simulink model "Powertrain_Performance_Design"  (R2024a)
settings: Solver=ode4  StartTime=0.0  StopTime=simtime  FixedStep=1  MaxStep=0.1  RelTol=1e-3
model workspace (MAT data in the model file):
  A_max = 2.22
  C_d = 0.23
  C_r = 0.011
  Cpack = 216
  DOD = [0 0.1 0.2 0.3 0.4 0.5 0.6 0.7 0.8 0.9 1 1.1 ... (1001 elements, 1001x1)]
  EM_N = [0 100 200 300 400 500 600 700 800 900 1000 1100 ... (171 elements, 1x171)]
  EM_N_Max = 17000
  EM_N_Min = 0
  EM_eff : Simulink.Parameter (value not decoded)
  Ff_N = 10218
  Kd = 0.3
  Ki = 0.02
  Kp = 15
  N_EM_eff = [0 34.06813627 68.13627255 102.2044088 136.2725451 170.3406814 204.4088176 238.4769539 272.5450902 306.6132265 340.6813627 374.749499 ... (500 elements, 1x500)]
  T_EM_Cont = [181.43664 181.43664 181.43664 181.43664 181.43664 181.43664 181.43664 181.43664 181.43664 181.43664 181.43664 181.43664 ... (171 elements, 171x1)]
  T_EM_Max = 375
  T_EM_Min = -375
  T_EM_Peak = [375 375 375 375 375 375 375 375 375 375 375 375 ... (171 elements, 171x1)]
  Tq_EM_eff = [0 0.751503006 1.503006012 2.254509018 3.006012024 3.75751503 4.509018036 5.260521042 6.012024048 6.763527054 7.51503006 8.266533066 ... (500 elements, 1x500)]
  Upack = [405.9 404.506 403.17334 401.89932 400.68136 399.51699 398.40386 397.33971 396.32239 395.34983 394.42006 393.53121 ... (1001 elements, 1001x1)]
  Upack_max = 405.9
  Vmax = 250
  a_r = 1.202
  eta_pack = 0.97
  eta_tr = 0.95
  g = 9.81
  ix = 9
  lambda_m = 1.05
  m_v = 1862
  r_w = 0.3277
  t_cool = 250
  t_peak = 20
values from neighbouring files (symbols this model uses):
  EM_eff = [78 78 78 78 78 78 78 78 78 78 78 78 ... (250000 elements, 500x500)]    [EM_eff.mat]
undefined symbols (not defined in the file or in its folder): selection, Soc_init, theta
(part 2 of 2)

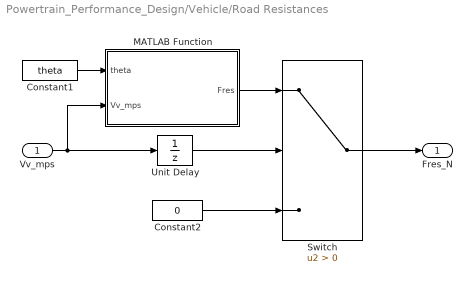
== system Powertrain_Performance_Design/Vehicle/Road Resistances ==
  Vv_mps : Inport
  Constant1 : Constant  Value=theta
  Constant2 : Constant  Value=0
  MATLAB Function : MATLAB Function  TreatAsAtomicUnit=on
  Switch : Switch  Criteria=u2 > Threshold  SaturateOnIntegerOverflow=off  InputSameDT=off
  Unit Delay : UnitDelay  SampleTime=-1  HasFrameUpgradeWarning=on
  Fres_N : Outport
  wires:
  Switch/1 -> Fres_N/1
  Unit Delay/1 -> Switch/2
  Vv_mps/1 -> MATLAB Function/2(Vv_mps), Unit Delay/1
  Constant1/1 -> MATLAB Function/1(theta)
  MATLAB Function/1(Fres) -> Switch/1
  Constant2/1 -> Switch/3

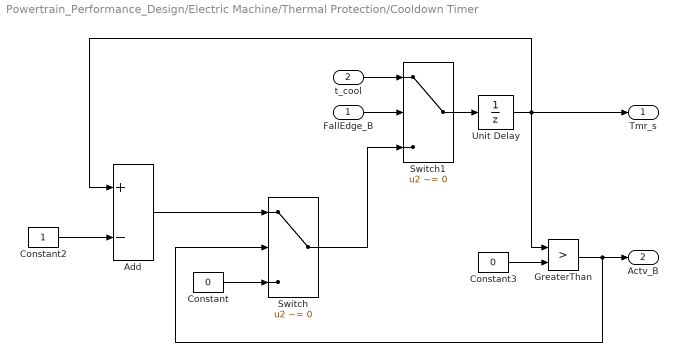
== system Powertrain_Performance_Design/Electric Machine/Thermal Protection/Cooldown Timer ==
  FallEdge_B : Inport
  t_cool : Inport  Port=2
  Add : Sum  Inputs=+-
  Constant : Constant  Value=0
  Constant2 : Constant
  Constant3 : Constant  Value=0
  GreaterThan : RelationalOperator  Operator=>  OutDataTypeStr=boolean  RndMeth=Simplest  InputSameDT=off
  Switch : Switch  Criteria=u2 ~= 0  SaturateOnIntegerOverflow=off  InputSameDT=off
  Switch1 : Switch  Criteria=u2 ~= 0  SaturateOnIntegerOverflow=off  InputSameDT=off
  Unit Delay : UnitDelay  SampleTime=-1  HasFrameUpgradeWarning=on
  Tmr_s : Outport
  Actv_B : Outport  Port=2
  wires:
  Add/1 -> Switch/1
  Constant/1 -> Switch/3
  GreaterThan/1 -> Actv_B/1, Switch/2
  Unit Delay/1 -> Tmr_s/1, Add/1, GreaterThan/1
  Constant3/1 -> GreaterThan/2
  Switch1/1 -> Unit Delay/1
  Constant2/1 -> Add/2
  t_cool/1 -> Switch1/1
  FallEdge_B/1 -> Switch1/2
  Switch/1 -> Switch1/3

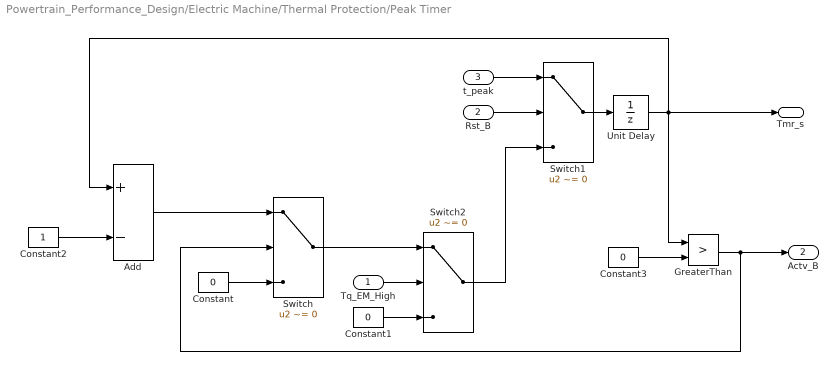
== system Powertrain_Performance_Design/Electric Machine/Thermal Protection/Peak Timer ==
  Tq_EM_High : Inport
  Rst_B : Inport  Port=2
  t_peak : Inport  Port=3
  Add : Sum  Inputs=+-
  Constant : Constant  Value=0
  Constant1 : Constant  Value=0
  Constant2 : Constant
  Constant3 : Constant  Value=0
  GreaterThan : RelationalOperator  Operator=>  OutDataTypeStr=boolean  RndMeth=Simplest  InputSameDT=off
  Switch : Switch  Criteria=u2 ~= 0  SaturateOnIntegerOverflow=off  InputSameDT=off
  Switch1 : Switch  Criteria=u2 ~= 0  SaturateOnIntegerOverflow=off  InputSameDT=off
  Switch2 : Switch  Criteria=u2 ~= 0  SaturateOnIntegerOverflow=off  InputSameDT=off
  Unit Delay : UnitDelay  SampleTime=-1  HasFrameUpgradeWarning=on
  Tmr_s : Outport
  Actv_B : Outport  Port=2
  wires:
  Rst_B/1 -> Switch1/2
  Constant1/1 -> Switch2/3
  Constant2/1 -> Add/2
  Switch/1 -> Switch2/1
  Add/1 -> Switch/1
  Tq_EM_High/1 -> Switch2/2
  t_peak/1 -> Switch1/1
  Constant3/1 -> GreaterThan/2
  Unit Delay/1 -> Tmr_s/1, Add/1, GreaterThan/1
  Switch2/1 -> Switch1/3
  GreaterThan/1 -> Switch/2, Actv_B/1
  Switch1/1 -> Unit Delay/1
  Constant/1 -> Switch/3

== system Powertrain_Performance_Design/Electric Machine/Thermal Protection/Subsystem ==
  Sig_Dec : Inport
  GreaterThan : RelationalOperator  Operator=>  OutDataTypeStr=boolean  RndMeth=Simplest  InputSameDT=off
  Unit Delay : UnitDelay  SampleTime=-1  HasFrameUpgradeWarning=on
  RisingEdge_B : Outport
  wires:
  Sig_Dec/1 -> Unit Delay/1, GreaterThan/1
  GreaterThan/1 -> RisingEdge_B/1
  Unit Delay/1 -> GreaterThan/2

== system Powertrain_Performance_Design/Electric Machine/Thermal Protection/Subsystem1 ==
  Sig_Dec : Inport
  GreaterThan : RelationalOperator  Operator=<  OutDataTypeStr=boolean  RndMeth=Simplest  InputSameDT=off
  Unit Delay : UnitDelay  SampleTime=-1  HasFrameUpgradeWarning=on
  FallEdge_B : Outport
  wires:
  GreaterThan/1 -> FallEdge_B/1
  Sig_Dec/1 -> Unit Delay/1, GreaterThan/1
  Unit Delay/1 -> GreaterThan/2

== system Powertrain_Performance_Design/Electric Machine/Thermal Protection/Subsystem2 ==
  Sig_Dec : Inport
  GreaterThan : RelationalOperator  Operator=<  OutDataTypeStr=boolean  RndMeth=Simplest  InputSameDT=off
  Unit Delay : UnitDelay  SampleTime=-1  HasFrameUpgradeWarning=on
  FallEdge_B : Outport
  wires:
  GreaterThan/1 -> FallEdge_B/1
  Sig_Dec/1 -> Unit Delay/1, GreaterThan/1
  Unit Delay/1 -> GreaterThan/2

== matlab function Powertrain_Performance_Design/Vehicle/Road Resistances/MATLAB Function ==
  data: theta input; Vv_mps input; Fres output
function Fres = Fres_calc(theta,Vv_mps)
m_v = 1862;
g = 9.81;
C_r = 0.011;
A_max = 2.22;
a_r = 1.202;
C_d = 0.23;

Fs = m_v*g*sind(theta);
Fr = m_v*g*C_r*cosd(theta);
Fa = 0.5*A_max*a_r*C_d*(Vv_mps)^2;

Fres = Fs+Fr+Fa;
end
